simulink model "testNoCopy"  (R2015a)
settings: Solver=ode3  StartTime=0.0  StopTime=Inf  FixedStep=0.001  RelTol=1e-3
libraries: xpcnetworkbufferlib x3, slrtlib x2
settings Model: xpc_rtwmakecfg_data=_xpcnblib_  Creator=djoshea  LastModifiedBy=djoshea
settings SolverCC: EnableConcurrentExecution=on
settings OptimizationCC: BlockReduction=off  OptimizeBlockIOStorage=off  BufferReuse=off  GlobalBufferReuse=off  ExpressionFolding=off  LocalBlockOutputs=off
settings HardwareCC: ProdIntDivRoundTo=Zero  ProdEndianess=LittleEndian  ProdLongLongMode=on  ProdHWDeviceType=Generic->32-bit x86 compatible
settings RTWCC: SystemTargetFile=slrt.tlc  TemplateMakefile=slrt_default_tmf  Description=Simulink Real-Time  GenerateReport=on  LaunchReport=on  RTWCompilerOptimization=on
settings CodeAppCC: MATLABSourceComments=on
settings SimulinkRealTimeCC: GeneratePreprocessorConditionals=Disable all  xPCisDownloadable=off

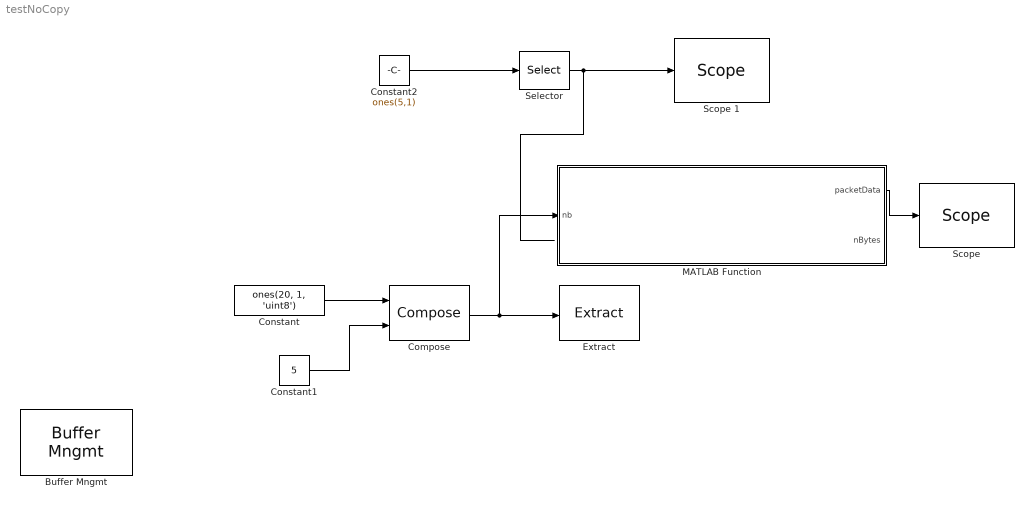
== system testNoCopy ==
  "Buffer Mngmt " : xpcnetworkbufferlib/Buffer Mngmt   Priority=-1  SampleTime=-1  PoolSizes=[100 10 10 200]  ShowTune=off
  "Compose " : xpcnetworkbufferlib/Compose 
  Constant : Constant  Value=ones(20, 1, 'uint8')
  Constant1 : Constant  Value=5
  Constant2 : Constant  Value=ones(5,1)
  "Extract " : xpcnetworkbufferlib/Extract   PacketSize=-1
  MATLAB Function : MATLAB Function  TreatAsAtomicUnit=on
  "Scope " : slrtlib/Displays and Logging/Scope   scopeno=1  scopetype=Target  autostart=on  viewmode=Graphical redraw  formatstr='%15.6f'  grid=on  ylimits=[0,0]  nosamples=250  noprepostsamples=0  interleave=1  triggermode=FreeRun  triggersignal=1  trigsignalfromport=off  triggerlevel=0.0  triggerslope=Either  triggerscope=1  triggersample=0  filename=data.dat  mode=Lazy  writesize=512  autorestart=off  dynamicfilemode=off  maxwritefilesize=512*1024^2
  Scope 1 : slrtlib/Displays and Logging/Scope   scopeno=2  scopetype=Target  autostart=on  viewmode=Graphical redraw  formatstr='%15.6f'  grid=on  ylimits=[0,0]  nosamples=250  noprepostsamples=0  interleave=1  triggermode=FreeRun  triggersignal=1  trigsignalfromport=off  triggerlevel=0.0  triggerslope=Either  triggerscope=1  triggersample=0  filename=data.dat  mode=Lazy  writesize=512  autorestart=off  dynamicfilemode=off  maxwritefilesize=512*1024^2
  Selector : Selector  InputPortWidth=5  Indices=[1 2 3 4]
  wires:
  "Compose "/1 -> MATLAB Function/1(nb), "Extract "/1
  Constant/1 -> "Compose "/1
  Constant1/1 -> "Compose "/2
  MATLAB Function/1(packetData) -> "Scope "/1
  Constant2/1 -> Selector/1
  Selector/1 -> Scope 1/1

== matlab function testNoCopy/MATLAB Function ==
  data: nb input; packetData output; nBytes output
function [packetData, nBytes] = accessPacket(nb)
%#codegen
    coder.cinclude('C:\Program Files\MATLAB\R2015a\toolbox\rtw\targets\xpc\target\build\xpcblocks\include\nblib.h');
    
    % nb is array of uint32
    buffer = coder.opaque('xpcNB*', 'NULL');
    buffer = cast(nb, 'like', buffer);

    dataPtr = coder.opaque('uint8_T*', 'NULL');
    dataPtr = coder.ceval('xpcNBData', buffer);
    
    nBytes = uint32(0);
    nBytes = coder.ceval('xpcNBBytes', buffer);
    
    nBytes = uint8(dataPtr + 1);

    packetData = coder.nullcopy(zeros(1500,1,'uint8'));
    nsizet = cast(1500,'like',coder.opaque('size_t','0'));
    coder.ceval('memcpy', coder.wref(packetData), dataPtr, nsizet);
    
end
